simulink model "outputFeedbackCtrl_constRef"  (R2022b)
settings: Solver=VariableStepAuto  StartTime=0.0  StopTime=70  RelTol=1e-3
values from neighbouring files (symbols this model uses):
  A = zeros(6,6)    [sim1_PartD.m]    (also in sim2_PartF.m; sim3_partG_part1.m; sim4_partG_part2.m)
  Bd = eye(6)    [sim3_partG_part1.m]    (also in sim4_partG_part2.m)
  Bk = [0,1/M,0,-1/M/l1,0,-1/M/l2]'    [sim3_partG_part1.m]    (also in sim4_partG_part2.m)
  C = zeros(3,6)    [sim1_PartD.m]    (also in sim2_PartF.m = [1,0,0,0,0,0; sim3_partG_part1.m = CC(var_sel,:); sim4_partG_part2.m = CC(var_sel,:))
  D = zeros(3,1)    [sim1_PartD.m]    (also in sim2_PartF.m = zeros(size(C,1),1); sim3_partG_part1.m = zeros(n_output_var,1); sim4_partG_part2.m = zeros(n_output_var,1))
  init_state = [x0,xd0,theta1_0,theta1_d0,theta2_0,theta2_d0]'    [sim1_PartD.m]    (also in sim2_PartF.m = [5,-0.5,20/180*pi,-0.5,-20/180*pi,0.5]'; sim3_partG_part1.m = [5,-0.5,20/180*pi,-0.5,-20/180*pi,0.5]'; sim4_partG_part2.m = [0,0,0,0,0,0]')
  K1 = K_bar(1:6)    [sim4_partG_part2.m]
  K2 = K_bar(7:end)    [sim4_partG_part2.m]
  L = LT'    [sim2_PartF.m]    (also in sim3_partG_part1.m = P*C'*sigma_v_inv; sim4_partG_part2.m = P*C'*sigma_v_inv)
  nc = length(sel_integral)    [sim4_partG_part2.m]
  S = II(sel_integral,:)    [sim4_partG_part2.m]
  u_disturb = u_disturb_list(i)    [sim4_partG_part2.m]
  u_inf = 0    [sim4_partG_part2.m]
  wn_Ts = 0.01    [sim3_partG_part1.m]    (also in sim4_partG_part2.m)
  xd = [10,0,0,0,0,0]'    [sim4_partG_part2.m]
libraries: simulink x2
settings Model: Creator=liuji  LastModifiedBy=liuji

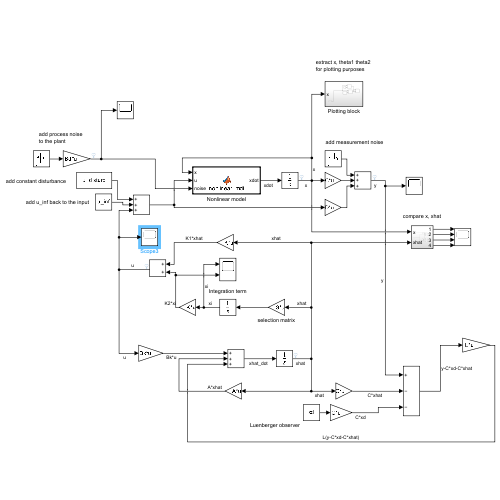
[thumbnail: Simulink's stored preview of the top-level diagram]
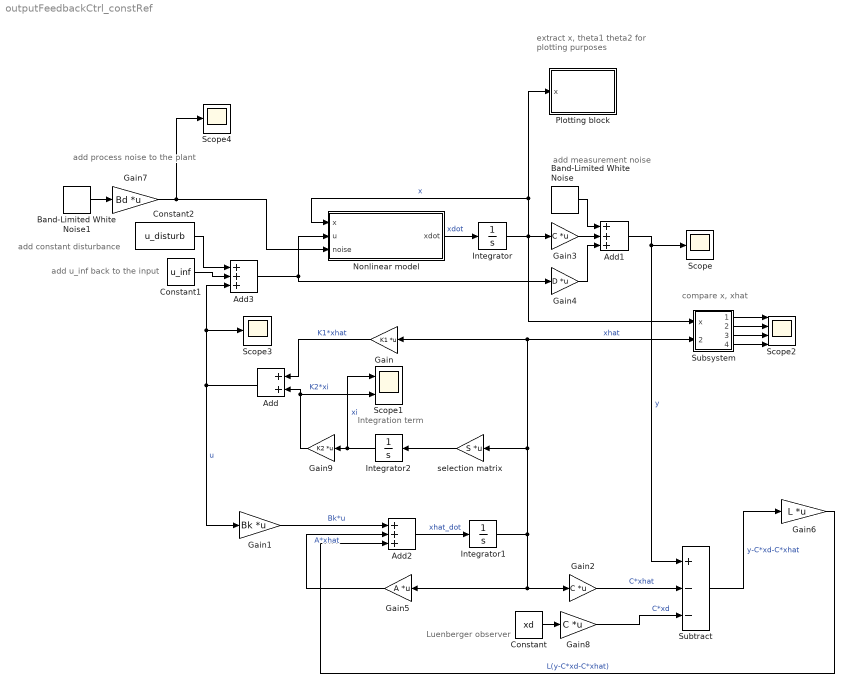
== system outputFeedbackCtrl_constRef ==
  note: add u_inf back to the input
  note: Integration term
  note: add measurement noise
  note: compare x, xhat
  note: add process noise
      | to the plant
  note: Luenberger observer
  note: extract x, theta1 theta2
      | for plotting purposes
  note: add constant disturbance
  Add : Sum
  Add1 : Sum  Inputs=+++
  Add2 : Sum  Inputs=+++
  Add3 : Sum  Inputs=+++
  Band-Limited White Noise : simulink/Sources/Band-Limited White Noise  Cov=wn_pow_measurement_vec  Ts=wn_Ts  seed=wn_measurement_seed
  Band-Limited White Noise1 : simulink/Sources/Band-Limited White Noise  Cov=wn_pow_process_vec  Ts=wn_Ts  seed=wn_process_seed
  Constant : Constant  Value=xd
  Constant1 : Constant  Value=u_inf
  Constant2 : Constant  Value=u_disturb
  Gain : Gain  Gain=K1  Multiplication=Matrix(K*u)
  Gain1 : Gain  Gain=Bk  Multiplication=Matrix(K*u)
  Gain2 : Gain  Gain=C  Multiplication=Matrix(K*u)
  Gain3 : Gain  Gain=C  Multiplication=Matrix(K*u)
  Gain4 : Gain  Gain=D  Multiplication=Matrix(K*u)
  Gain5 : Gain  Gain=A  Multiplication=Matrix(K*u)
  Gain6 : Gain  Gain=L  Multiplication=Matrix(K*u)
  Gain7 : Gain  Gain=Bd  Multiplication=Matrix(K*u)
  Gain8 : Gain  Gain=C  Multiplication=Matrix(K*u)
  Gain9 : Gain  Gain=K2  Multiplication=Matrix(K*u)
  Integrator : Integrator  InitialCondition=init_state
  Integrator1 : Integrator  InitialCondition=[0,0,0,0,0,0]'
  Integrator2 : Integrator  InitialCondition=zeros(nc,1)
  Nonlinear model : MATLAB Function  TreatAsAtomicUnit=on
  Plotting block : Subsystem
  Scope : Scope
  Scope1 : Scope  NumInputPorts=2
  Scope2 : Scope  NumInputPorts=4
  Scope3 : Scope
  Scope4 : Scope
  Subsystem : Subsystem
  Subtract : Sum  Inputs=+--
  selection matrix : Gain  Gain=S  Multiplication=Matrix(K*u)
  wires:
  Integrator/1 -> Plotting block/1(x), Nonlinear model/1(x), Subsystem/1(x), Gain3/1  "x"
  Nonlinear model/1(xdot) -> Integrator/1  "xdot"
  Gain1/1 -> Add2/1  "Bk*u"
  Add1/1 -> Scope/1, Subtract/1  "y"
  Integrator1/1 -> selection matrix/1, Gain/1, Subsystem/2(xhat), Gain2/1, Gain5/1  "xhat"
  Add2/1 -> Integrator1/1  "xhat_dot"
  Gain5/1 -> Add2/2  "A*xhat"
  Gain2/1 -> Subtract/2  "C*xhat"
  Subtract/1 -> Gain6/1  "y-C*xd-C*xhat"
  Gain6/1 -> Add2/3  "L(y-C*xd-C*xhat)"
  Gain/1 -> Add/1  "K1*xhat"
  Band-Limited White Noise1/1 -> Gain7/1
  Gain4/1 -> Add1/3
  Gain3/1 -> Add1/2
  Band-Limited White Noise/1 -> Add1/1
  Gain7/1 -> Nonlinear model/3(noise), Scope4/1
  Subsystem/1(Out1) -> Scope2/1
  Subsystem/2(Out2) -> Scope2/2
  Subsystem/3(Outport) -> Scope2/3
  Subsystem/4(Outport1) -> Scope2/4
  Constant/1 -> Gain8/1
  Gain8/1 -> Subtract/3  "C*xd"
  selection matrix/1 -> Integrator2/1
  Integrator2/1 -> Scope1/1, Gain9/1  "xi"
  Gain9/1 -> Add/2, Scope1/2  "K2*xi"
  Add/1 -> Gain1/1, Scope3/1, Add3/3  "u"
  Add3/1 -> Gain4/1, Nonlinear model/2(u)
  Constant1/1 -> Add3/2
  Constant2/1 -> Add3/1

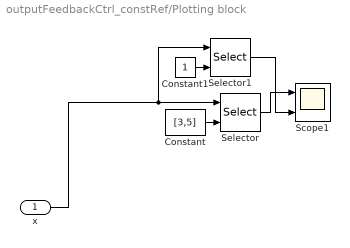
== system outputFeedbackCtrl_constRef/Plotting block ==
  x : Inport
  Constant : Constant  Value=[3,5]
  Constant1 : Constant
  Scope1 : Scope  NumInputPorts=2
  Selector : Selector  InputPortWidth=6  IndexOptions=Index vector (port)  Indices=[1 3]  OutputSizes=1
  Selector1 : Selector  InputPortWidth=6  IndexOptions=Index vector (port)  Indices=[1 3]  OutputSizes=1
  wires:
  Selector1/1 -> Scope1/2
  x/1 -> Selector1/1, Selector/1
  Selector/1 -> Scope1/1
  Constant1/1 -> Selector1/2
  Constant/1 -> Selector/2

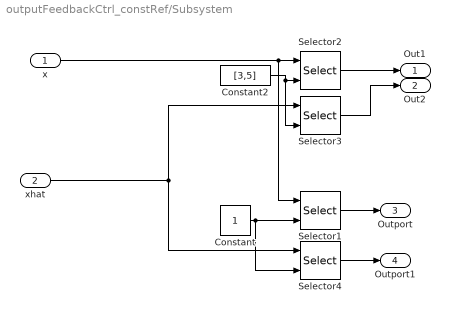
== system outputFeedbackCtrl_constRef/Subsystem ==
  x : Inport
  xhat : Inport  Port=2
  Constant : Constant
  Constant2 : Constant  Value=[3,5]
  Selector{1..4} (4 alike) : Selector  InputPortWidth=6  IndexOptions=Index vector (port)  Indices=[1 3]  OutputSizes=1
  Out1 : Outport
  Out2 : Outport  Port=2
  Outport : Outport  Port=3
  Outport1 : Outport  Port=4
  wires:
  xhat/1 -> Selector4/1, Selector3/1
  Constant2/1 -> Selector3/2, Selector2/2
  Selector2/1 -> Out1/1
  x/1 -> Selector2/1, Selector1/1
  Selector3/1 -> Out2/1
  Constant/1 -> Selector4/2, Selector1/2
  Selector4/1 -> Outport1/1
  Selector1/1 -> Outport/1

== matlab function outputFeedbackCtrl_constRef/Nonlinear model ==
  data: x input; u input; noise input; xdot output; param parameter
function xdot = nonlinear_mdl(x,u,noise,param)
    % implements the original dyanmics model
    M = param.M;
    m1 = param.m1;
    m2 = param.m2;
    l1 = param.l1;
    l2 = param.l2;
    g = param.g;
    x1 = x(1);
    x2 = x(2);
    x3 = x(3);
    x4 = x(4);
    x5 = x(5);
    x6 = x(6);
    xdot = zeros(6,1);
    xdot(1) = x2;
    xdot(2) = 1/(M + m1*sin(x3)^2 + m2*sin(x5)^2)*...
        (m1*g*sin(x3)*cos(x3) + m1*l1*x4^2*sin(x3) + m2*g*sin(x5)*cos(x5) + m2*l2*x6^2*sin(x5) + u);
    xdot(3) = x4;
    xdot(4) = -1/(l1*( M + m1*sin(x3)^2 + m2*sin(x5)^2 ))*...
        (m1*g*sin(x3) + m2*g*sin(x5)*cos(x3-x5) + m1*l1*x4^2*sin(x3)*cos(x3) + m2*l2*x6^2*sin(x5)*cos(x3) + ...
        M*g*sin(x3) + u*cos(x3));
    xdot(5) = x6;
    xdot(6) = -1/(l2*( M + m1*sin(x3)^2 + m2*sin(x5)^2 ))*...
        (m2*g*sin(x5) + m1*g*sin(x3)*cos(x3-x5) + m1*l1*x4^2*sin(x3)*cos(x5) + m2*l2*x6^2*sin(x5)*cos(x5) + ...
        M*g*sin(x5) + u*cos(x5));
    % add process noise
    xdot = xdot + noise;
